simulink model "Simulink_with_unkown_parameters_case"  (R2020b)
settings: Solver=FixedStepAuto  StartTime=0.0  StopTime=50  FixedStep=0.001  MaxStep=0.01  RelTol=1e-9
values from neighbouring files (symbols this model uses):
  A0 = [30 3;3 30]    [Main_with_unkown_parameters_case.m]
  A1 = [30 3;3 30]    [Main_with_unkown_parameters_case.m]
  A2 = [10 1;1 10]    [Main_with_unkown_parameters_case.m]
  AE = blkdiag([0 pi/2;-pi/2 0],[0 pi/2;-pi/2 0])    [Main.m]    (also in Main_with_unkown_parameters_case.m)
  AM = blkdiag([0 1;-1 0],[0 1;-1 0])    [Main.m]    (also in Main_with_unkown_parameters_case.m)
  dq1_0 = [0;0]    [Main.m]    (also in Main_with_unkown_parameters_case.m)
  dq2_0 = [0;0]    [Main.m]    (also in Main_with_unkown_parameters_case.m)
  dq3_0 = [0;0]    [Main.m]    (also in Main_with_unkown_parameters_case.m)
  dq4_0 = [0;0]    [Main.m]    (also in Main_with_unkown_parameters_case.m)
  GammaE = blkdiag([1 0],[1 0])    [Main.m]    (also in Main_with_unkown_parameters_case.m)
  GammaM = blkdiag([1 0],[1 0])    [Main.m]    (also in Main_with_unkown_parameters_case.m)
  kapa = 100    [Main_with_unkown_parameters_case.m]
  Kd = 600    [Main.m]    (also in Main_with_unkown_parameters_case.m)
  Kp = 800    [Main.m]    (also in Main_with_unkown_parameters_case.m)
  l1 = 1.5    [Main.m]    (also in Main_with_unkown_parameters_case.m)
  l2 = 1.5    [Main.m]    (also in Main_with_unkown_parameters_case.m)
  M0 = [p1+p2+p4,p2;p2,p2+p5]+[2*p3,p3;p3,0]*cos(0)*0.5    [Main_with_unkown_parameters_case.m]
  N = 100    [Main_with_unkown_parameters_case.m]
  ON_OFF = 0    [Main.m]    (also in Main_with_unkown_parameters_case.m)
  p1 = m1*lc1^2+m2*l1^2+2*m2*l1*lc2^2+I1    (= 4.8375)    [Main.m]    (also in Main_with_unkown_parameters_case.m)
  p10 = 0    [Main.m]    (also in Main_with_unkown_parameters_case.m)
  p2 = m2*lc2^2+I2    (= 0.75)    [Main.m]    (also in Main_with_unkown_parameters_case.m)
  p3 = m2*l1*lc2    (= 1.125)    [Main.m]    (also in Main_with_unkown_parameters_case.m)
  p4 = 0    [Main.m]    (also in Main_with_unkown_parameters_case.m)
  p5 = 0    [Main.m]    (also in Main_with_unkown_parameters_case.m)
  p6 = (m1*lc1+m2*l1)*g    (= 23.544)    [Main.m]    (also in Main_with_unkown_parameters_case.m)
  p7 = m2*lc2*g    (= 7.3575)    [Main.m]    (also in Main_with_unkown_parameters_case.m)
  p8 = m2*lc2    (= 0.75)    [Main.m]    (also in Main_with_unkown_parameters_case.m)
  p9 = 0    [Main.m]    (also in Main_with_unkown_parameters_case.m)
  q1_0 = [-0.1;pi/3+0.2]    [Main.m]    (also in Main_with_unkown_parameters_case.m)
  q2_0 = [pi/2;2*pi/3]    [Main.m]    (also in Main_with_unkown_parameters_case.m)
  q3_0 = [pi-0.2;pi/3+0.2]    [Main.m]    (also in Main_with_unkown_parameters_case.m)
  q4_0 = [0.2;-pi/3-0.2]    [Main.m]    (also in Main_with_unkown_parameters_case.m)
  x1_0 = [0;0]    [Main.m]    (also in Main_with_unkown_parameters_case.m)
  x2_0 = [5;0]    [Main.m]    (also in Main_with_unkown_parameters_case.m)
  x3_0 = [5;3]    [Main.m]    (also in Main_with_unkown_parameters_case.m)
  x4_0 = [0;3]    [Main.m]    (also in Main_with_unkown_parameters_case.m)
(part 2 of 2)

== system Simulink_with_unkown_parameters_case/planar 3/Jacobian matrix ==
  q : Inport
  Demux : Demux  Outputs=2
  Gain : Gain  Gain=-l1
  Gain1 : Gain  Gain=-l2
  Gain2 : Gain  Gain=l1
  Gain3 : Gain  Gain=l2
  Sum : Sum  Inputs=++|
  Sum1 : Sum  Inputs=|++
  Sum2 : Sum  Inputs=|++
  Trigonometric Function : Trigonometry
  Trigonometric Function1 : Trigonometry
  Trigonometric Function2 : Trigonometry  Operator=cos
  Trigonometric Function3 : Trigonometry  Operator=cos
  Vector Concatenate : Concatenate  Mode=Multidimensional array  ConcatenateDimension=2
  Vector Concatenate1 : Concatenate  Mode=Multidimensional array  ConcatenateDimension=2
  Vector Concatenate2 : Concatenate  Mode=Multidimensional array
  J(q) : Outport
  wires:
  Vector Concatenate2/1 -> J(q)/1
  Vector Concatenate/1 -> Vector Concatenate2/2
  Vector Concatenate1/1 -> Vector Concatenate2/1
  Sum2/1 -> Vector Concatenate/1  "J21"
  Sum1/1 -> Vector Concatenate1/1  "J11"
  Gain3/1 -> Vector Concatenate/2, Sum2/2  "J22"
  Gain2/1 -> Sum2/1
  Gain/1 -> Sum1/1
  Gain1/1 -> Sum1/2, Vector Concatenate1/2  "J12"
  Trigonometric Function2/1 -> Gain2/1
  Trigonometric Function3/1 -> Gain3/1
  Trigonometric Function1/1 -> Gain1/1
  Sum/1 -> Trigonometric Function3/1, Trigonometric Function1/1
  Demux/1 -> Trigonometric Function2/1, Trigonometric Function/1, Sum/1  "q1"
  Trigonometric Function/1 -> Gain/1
  Demux/2 -> Sum/2  "q2"
  q/1 -> Demux/1

== system Simulink_with_unkown_parameters_case/planar 3/Matrix C(q,dq)  ==
  q : Inport
  dq : Inport  Port=2
  Demux : Demux  Outputs=2
  Demux1 : Demux  Outputs=2
  Gain : Gain  Gain=[-p3,-p3;p3,0]
  Gain1 : Gain  Gain=[0,1;1,0]
  Gain2 : Gain  Gain=[1,0;0,0]
  Product : Product
  Sum : Sum
  Terminator : Terminator
  Trigonometric Function : Trigonometry
  Vector Concatenate : Concatenate  Mode=Multidimensional array
  Vector Concatenate1 : Concatenate  Mode=Multidimensional array  ConcatenateDimension=2
  C : Outport
  wires:
  Product/1 -> C/1
  Sum/1 -> Product/2
  Gain2/1 -> Sum/2
  Gain1/1 -> Sum/1
  Demux1/2 -> Gain2/1  "dq2"
  Demux1/1 -> Gain1/1  "dq1"
  dq/1 -> Demux1/1
  Gain/1 -> Product/1
  Trigonometric Function/1 -> Vector Concatenate/1, Vector Concatenate/2
  Vector Concatenate/1 -> Vector Concatenate1/2, Vector Concatenate1/1
  Demux/2 -> Trigonometric Function/1  "q2"
  Demux/1 -> Terminator/1
  Vector Concatenate1/1 -> Gain/1
  q/1 -> Demux/1

== system Simulink_with_unkown_parameters_case/planar 3/Matrix F ==
  Constant : Constant  Value=[p9,0;0,p10]
  F : Outport
  wires:
  Constant/1 -> F/1

== system Simulink_with_unkown_parameters_case/planar 3/Matrix G(q) ==
  q : Inport
  Demux : Demux  Outputs=2
  Gain : Gain  Gain=[p6,p7;0,p8]  Multiplication=Matrix(K*u)
  Mux : Mux  Inputs=2
  Sum : Sum  Inputs=++|
  Trigonometric Function : Trigonometry  Operator=cos
  Trigonometric Function1 : Trigonometry  Operator=cos
  G : Outport
  wires:
  Mux/1 -> Gain/1
  Trigonometric Function1/1 -> Mux/2
  Trigonometric Function/1 -> Mux/1
  Sum/1 -> Trigonometric Function1/1  "q1+q2"
  q/1 -> Demux/1
  Demux/1 -> Trigonometric Function/1, Sum/1  "q1"
  Demux/2 -> Sum/2  "q2"
  Gain/1 -> G/1

== system Simulink_with_unkown_parameters_case/planar 3/Matrix M(q)  ==
  q : Inport
  Constant : Constant  Value=[p1+p2+p4,p2;p2,p2+p5]
  Demux : Demux  Outputs=2
  Gain : Gain  Gain=[2*p3,p3;p3,0]
  Sum : Sum  Inputs=|++
  Terminator : Terminator
  Trigonometric Function : Trigonometry  Operator=cos
  Vector Concatenate : Concatenate  Mode=Multidimensional array
  Vector Concatenate1 : Concatenate  Mode=Multidimensional array  ConcatenateDimension=2
  M : Outport
  wires:
  q/1 -> Demux/1
  Vector Concatenate1/1 -> Gain/1
  Sum/1 -> M/1  "M"
  Demux/1 -> Terminator/1
  Demux/2 -> Trigonometric Function/1  "q2"
  Vector Concatenate/1 -> Vector Concatenate1/1, Vector Concatenate1/2
  Constant/1 -> Sum/1
  Trigonometric Function/1 -> Vector Concatenate/2, Vector Concatenate/1
  Gain/1 -> Sum/2

== system Simulink_with_unkown_parameters_case/planar 3/forward kinematics ==
  q : Inport
  Constant : Constant  Value=x0
  Demux : Demux  Outputs=2
  Gain : Gain  Gain=l1
  Gain1 : Gain  Gain=l2
  Gain2 : Gain  Gain=l1
  Gain3 : Gain  Gain=l2
  Mux : Mux  Inputs=2
  Sum : Sum  Inputs=++|
  Sum1 : Sum  Inputs=++|
  Sum2 : Sum  Inputs=|++
  Sum3 : Sum  Inputs=|++
  Trigonometric Function : Trigonometry  Operator=cos
  Trigonometric Function1 : Trigonometry  Operator=cos
  Trigonometric Function2 : Trigonometry
  Trigonometric Function3 : Trigonometry
  x : Outport
  wires:
  Constant/1 -> Sum3/2
  Sum3/1 -> x/1
  Sum2/1 -> Mux/2
  Sum1/1 -> Mux/1
  Gain3/1 -> Sum2/2
  Gain2/1 -> Sum2/1
  Gain/1 -> Sum1/1
  Gain1/1 -> Sum1/2
  Trigonometric Function2/1 -> Gain2/1
  Trigonometric Function3/1 -> Gain3/1
  Trigonometric Function1/1 -> Gain1/1
  Sum/1 -> Trigonometric Function3/1, Trigonometric Function1/1
  Demux/1 -> Trigonometric Function2/1, Trigonometric Function/1, Sum/1  "q1"
  Trigonometric Function/1 -> Gain/1
  Demux/2 -> Sum/2  "q2"
  Mux/1 -> Sum3/1
  q/1 -> Demux/1

== system Simulink_with_unkown_parameters_case/planar 4/Jacobian matrix ==
  q : Inport
  Demux : Demux  Outputs=2
  Gain : Gain  Gain=-l1
  Gain1 : Gain  Gain=-l2
  Gain2 : Gain  Gain=l1
  Gain3 : Gain  Gain=l2
  Sum : Sum  Inputs=++|
  Sum1 : Sum  Inputs=|++
  Sum2 : Sum  Inputs=|++
  Trigonometric Function : Trigonometry
  Trigonometric Function1 : Trigonometry
  Trigonometric Function2 : Trigonometry  Operator=cos
  Trigonometric Function3 : Trigonometry  Operator=cos
  Vector Concatenate : Concatenate  Mode=Multidimensional array  ConcatenateDimension=2
  Vector Concatenate1 : Concatenate  Mode=Multidimensional array  ConcatenateDimension=2
  Vector Concatenate2 : Concatenate  Mode=Multidimensional array
  J(q) : Outport
  wires:
  Vector Concatenate2/1 -> J(q)/1
  Vector Concatenate/1 -> Vector Concatenate2/2
  Vector Concatenate1/1 -> Vector Concatenate2/1
  Sum2/1 -> Vector Concatenate/1  "J21"
  Sum1/1 -> Vector Concatenate1/1  "J11"
  Gain3/1 -> Vector Concatenate/2, Sum2/2  "J22"
  Gain2/1 -> Sum2/1
  Gain/1 -> Sum1/1
  Gain1/1 -> Sum1/2, Vector Concatenate1/2  "J12"
  Trigonometric Function2/1 -> Gain2/1
  Trigonometric Function3/1 -> Gain3/1
  Trigonometric Function1/1 -> Gain1/1
  Sum/1 -> Trigonometric Function3/1, Trigonometric Function1/1
  Demux/1 -> Trigonometric Function2/1, Trigonometric Function/1, Sum/1  "q1"
  Trigonometric Function/1 -> Gain/1
  Demux/2 -> Sum/2  "q2"
  q/1 -> Demux/1

== system Simulink_with_unkown_parameters_case/planar 4/Matrix C(q,dq)  ==
  q : Inport
  dq : Inport  Port=2
  Demux : Demux  Outputs=2
  Demux1 : Demux  Outputs=2
  Gain : Gain  Gain=[-p3,-p3;p3,0]
  Gain1 : Gain  Gain=[0,1;1,0]
  Gain2 : Gain  Gain=[1,0;0,0]
  Product : Product
  Sum : Sum
  Terminator : Terminator
  Trigonometric Function : Trigonometry
  Vector Concatenate : Concatenate  Mode=Multidimensional array
  Vector Concatenate1 : Concatenate  Mode=Multidimensional array  ConcatenateDimension=2
  C : Outport
  wires:
  Product/1 -> C/1
  Sum/1 -> Product/2
  Gain2/1 -> Sum/2
  Gain1/1 -> Sum/1
  Demux1/2 -> Gain2/1  "dq2"
  Demux1/1 -> Gain1/1  "dq1"
  dq/1 -> Demux1/1
  Gain/1 -> Product/1
  Trigonometric Function/1 -> Vector Concatenate/1, Vector Concatenate/2
  Vector Concatenate/1 -> Vector Concatenate1/2, Vector Concatenate1/1
  Demux/2 -> Trigonometric Function/1  "q2"
  Demux/1 -> Terminator/1
  Vector Concatenate1/1 -> Gain/1
  q/1 -> Demux/1

== system Simulink_with_unkown_parameters_case/planar 4/Matrix F ==
  Constant : Constant  Value=[p9,0;0,p10]
  F : Outport
  wires:
  Constant/1 -> F/1

== system Simulink_with_unkown_parameters_case/planar 4/Matrix G(q) ==
  q : Inport
  Demux : Demux  Outputs=2
  Gain : Gain  Gain=[p6,p7;0,p8]  Multiplication=Matrix(K*u)
  Mux : Mux  Inputs=2
  Sum : Sum  Inputs=++|
  Trigonometric Function : Trigonometry  Operator=cos
  Trigonometric Function1 : Trigonometry  Operator=cos
  G : Outport
  wires:
  Mux/1 -> Gain/1
  Trigonometric Function1/1 -> Mux/2
  Trigonometric Function/1 -> Mux/1
  Sum/1 -> Trigonometric Function1/1  "q1+q2"
  q/1 -> Demux/1
  Demux/1 -> Trigonometric Function/1, Sum/1  "q1"
  Demux/2 -> Sum/2  "q2"
  Gain/1 -> G/1

== system Simulink_with_unkown_parameters_case/planar 4/Matrix M(q)  ==
  q : Inport
  Constant : Constant  Value=[p1+p2+p4,p2;p2,p2+p5]
  Demux : Demux  Outputs=2
  Gain : Gain  Gain=[2*p3,p3;p3,0]
  Sum : Sum  Inputs=|++
  Terminator : Terminator
  Trigonometric Function : Trigonometry  Operator=cos
  Vector Concatenate : Concatenate  Mode=Multidimensional array
  Vector Concatenate1 : Concatenate  Mode=Multidimensional array  ConcatenateDimension=2
  M : Outport
  wires:
  q/1 -> Demux/1
  Vector Concatenate1/1 -> Gain/1
  Sum/1 -> M/1  "M"
  Demux/1 -> Terminator/1
  Demux/2 -> Trigonometric Function/1  "q2"
  Vector Concatenate/1 -> Vector Concatenate1/1, Vector Concatenate1/2
  Constant/1 -> Sum/1
  Trigonometric Function/1 -> Vector Concatenate/2, Vector Concatenate/1
  Gain/1 -> Sum/2

== system Simulink_with_unkown_parameters_case/planar 4/forward kinematics ==
  q : Inport
  Constant : Constant  Value=x0
  Demux : Demux  Outputs=2
  Gain : Gain  Gain=l1
  Gain1 : Gain  Gain=l2
  Gain2 : Gain  Gain=l1
  Gain3 : Gain  Gain=l2
  Mux : Mux  Inputs=2
  Sum : Sum  Inputs=++|
  Sum1 : Sum  Inputs=++|
  Sum2 : Sum  Inputs=|++
  Sum3 : Sum  Inputs=|++
  Trigonometric Function : Trigonometry  Operator=cos
  Trigonometric Function1 : Trigonometry  Operator=cos
  Trigonometric Function2 : Trigonometry
  Trigonometric Function3 : Trigonometry
  x : Outport
  wires:
  Constant/1 -> Sum3/2
  Sum3/1 -> x/1
  Sum2/1 -> Mux/2
  Sum1/1 -> Mux/1
  Gain3/1 -> Sum2/2
  Gain2/1 -> Sum2/1
  Gain/1 -> Sum1/1
  Gain1/1 -> Sum1/2
  Trigonometric Function2/1 -> Gain2/1
  Trigonometric Function3/1 -> Gain3/1
  Trigonometric Function1/1 -> Gain1/1
  Sum/1 -> Trigonometric Function3/1, Trigonometric Function1/1
  Demux/1 -> Trigonometric Function2/1, Trigonometric Function/1, Sum/1  "q1"
  Trigonometric Function/1 -> Gain/1
  Demux/2 -> Sum/2  "q2"
  Mux/1 -> Sum3/1
  q/1 -> Demux/1

== matlab function Simulink_with_unkown_parameters_case/Distibuted control law ==
  data: x1 input size=2; e1_hat output size=2; x2 input size=2; x3 input size=2; x4 input size=2; e2_hat output size=2; e3_hat output size=2; e4_hat output size=2; B parameter
function [e1_hat,e2_hat,e3_hat,e4_hat] = fcn(x1,x2,x3,x4,B)
%%%%%%%%%%%%%%%%%%%%%%%%%%%%%%%%
%Graph of connections between agents is depicted below, where vertices are
%shown without brackets and links are referenced with brackets 
%                  2
%                 / \
%             (2)/   \(1)
%               /     \
%              3--(5)--1
%               \     /
%            (3) \   / (4)
%                 \ /
%                  4
%%%%%%%%%%%%%%%%%%%%%%%%%%%%%%%%
x=[x1',x2',x3',x4']';
B_bar=kron(B,eye(2));
z=B_bar'*x;
Dz=2*blkdiag(z(1:2),z(3:4),z(5:6),z(7:8),z(9:10));
e=z(1:2:10).^2+z(2:2:10).^2-[0.4;0.4;0.4;0.4;0.4*sqrt(2)].^2;
e_hat=B_bar*Dz*e;
e1_hat=e_hat(1:2);
e2_hat=e_hat(3:4);
e3_hat=e_hat(5:6);
e4_hat=e_hat(7:8);
